simulink model "AMC_BLDC"  (R2023a)
settings: Solver=FixedStepDiscrete  StartTime=0.0  StopTime=10.0  RelTol=1e-3  EnableMultiTasking=on
model workspace (MAT data in the model file):
  AMC_BLDC_Ts = Simulink.Parameter
  AMC_BLDC_Ts.Value = 0.001
  AMC_BLDC_Ts.DataType = 'auto'
  AMC_BLDC_Ts.DocUnits = 's'
  AMC_BLDC_Ts.Complexity = 'real'
  AMC_BLDC_Ts.Dimensions = [1 1]
  ControlFOC_Ts = Simulink.Parameter
  ControlFOC_Ts.Value = 3.65714285714e-05
  ControlFOC_Ts.DataType = 'auto'
  ControlFOC_Ts.DocUnits = 's'
  ControlFOC_Ts.Complexity = 'real'
  ControlFOC_Ts.Dimensions = [1 1]
settings Model: DataDictionary=EmbeddedBoardDD.sldd  Creator=upattacini  LastModifiedBy=mfussi
settings SolverCC: AllowMultiTaskInputOutput=on  ConcurrentTasks=on  AlgebraicLoopSolver=TrustRegion  AutoInsertRateTranBlk=on  InsertRTBMode=Never (minimum delay)
settings DataIOCC: SaveOutput=off  SignalLogging=off  DSMLogging=off  SaveTime=off  ReturnWorkspaceOutputs=off
settings OptimizationCC: DefaultParameterBehavior=Inlined  DefaultUnderspecifiedDataType=single  StrengthReduction=on  PassReuseOutputArgsAs=Individual arguments  ZeroExternalMemoryAtStartup=off  ZeroInternalMemoryAtStartup=off  OptimizeBlockOrder=speed  OptimizationPriority=Speed  OptimizationCustomize=off  MultiThreadedLoops=on  EfficientTunableParamExpr=on
settings DebuggingCC: ParameterPrecisionLossMsg=none  UnconnectedInputMsg=warning  UnconnectedOutputMsg=warning  UnconnectedLineMsg=warning
settings HardwareCC: ProdBitPerPointer=32  ProdBitPerSizeT=32  ProdBitPerPtrDiffT=32  ProdLargestAtomicInteger=Long  ProdLargestAtomicFloat=Double  ProdWordSize=32  ProdHWDeviceType=ARM Compatible->ARM Cortex-M
settings ModelReferenceCC: UpdateModelReferenceTargets=Force  EnableRefExpFcnMdlSchedulingChecks=on  ModelReferenceNumInstancesAllowed=Single
settings SFSimCC: MATLABDynamicMemAlloc=off
settings RTWCC: Description=Embedded Coder  SystemTargetFile=ert.tlc  GenCodeOnly=on  PackageGeneratedCodeAndArtifacts=on  PackageName=AMC_BLDC  TemplateMakefile=ert_default_tmf  TargetLang=C++  DLArmComputeVersion=19.05
settings CodeAppCC: ForceParamTrailComments=on  IgnoreCustomStorageClasses=off  MaxIdLength=60  OperatorAnnotations=on  SimulinkDataObjDesc=on  SFDataObjDesc=on  InsertBlockDesc=on
settings ERTTargetCC: TargetLangStandard=C++03 (ISO)  CodeReplacementLibrary=ARM Cortex-M,iCubTech  GenerateSampleERTMain=on  InlinedParameterPlacement=NonHierarchical  TargetOS=NativeThreadsExample  RootIOFormat=Structure reference  ERTCustomFileTemplate=example_file_process.tlc

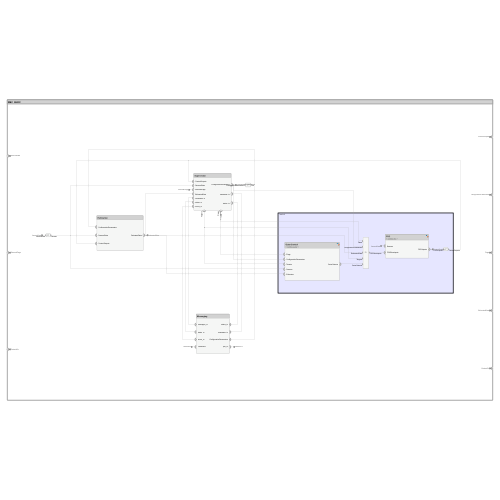
[thumbnail: Simulink's stored preview of the top-level diagram]
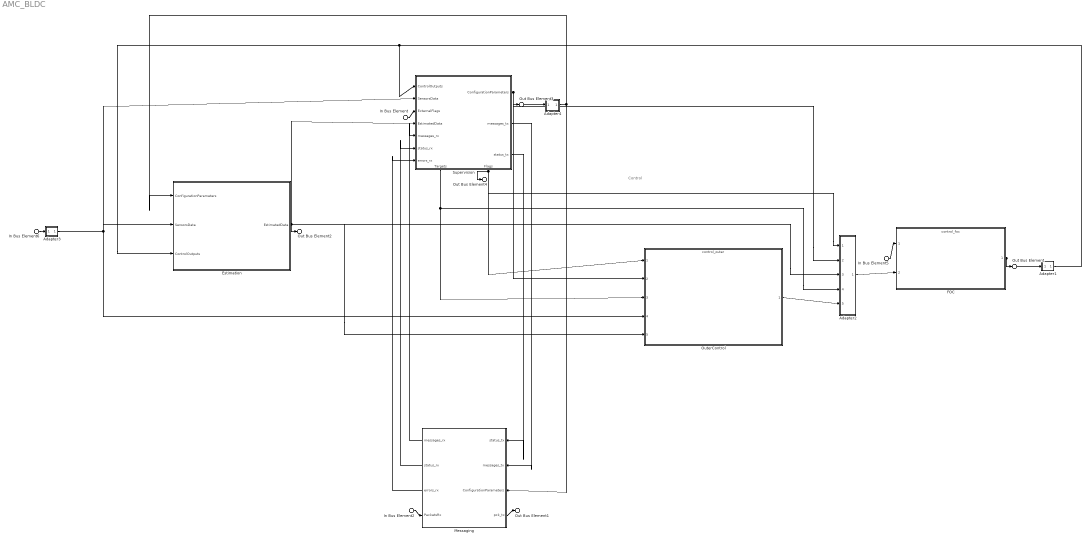
== system AMC_BLDC ==
  note: Control
  In Bus Element5 : Inport  PortName=SensorsData
  In Bus Element6 : Inport  PortName=SensorsData
  In Bus Element : Inport  Port=2  PortName=ExternalFlags
  In Bus Element2 : Inport  Port=3  PortName=PacketsRx
  Adapter1 : Subsystem
      settings: PortSchema="{\"entries\":[{\"content\":{\"margin\":10,\"minimumSpacing\":15,\"sides\":[{\"content\":{\"connectorIds\":[\"In1\"]},\"type\":\"ConnectorPlacement.EquallySpacedRectSide\",\"uuid\":\"3636cd8d-cbd3-4f3a-bfc2-0b6f64e30752\"},{\"content\":{\"connectorIds\":[\"Out1\"],\"side\":\"RIGHT\"},\"type\":\"ConnectorPlacement.EquallySpacedRectSide\",\"uuid\":\"432d5fc1-0f50-4fcc-8edd-5172f2fe1fb1\"},{\"content\":{\"connectorIds\":[],\"side\":\"TOP\"},\"type\":\"ConnectorPlacement.EquallySpacedRectSide\",\"uuid\":\"ba372e81-7918-4711-815e-6864fd5d6a77\"}]},\"type\":\"ConnectorPlacement.EquallySpacedConnector\",\"uuid\":\"ce9b4e59-ddcd-4a55-aad5-bd568399e791\"}],\"packageUris\":[\"http://schema.mathworks.com/mf0/Connector/R2020b\"],\"version\":\"1.0\"}"
  Adapter2 : Subsystem
      settings: PortSchema="{\"entries\":[{\"content\":{\"margin\":10,\"minimumSpacing\":15,\"sides\":[{\"content\":{\"connectorIds\":[\"In1\",\"In2\",\"In3\",\"In4\",\"In5\"]},\"type\":\"ConnectorPlacement.EquallySpacedRectSide\",\"uuid\":\"eaff3585-0474-4235-a4f6-c3e0d182b6aa\"},{\"content\":{\"connectorIds\":[\"Out1\"],\"side\":\"RIGHT\"},\"type\":\"ConnectorPlacement.EquallySpacedRectSide\",\"uuid\":\"c828b82e-1a15-4cb3-9e29-bf61868b0eb2\"},{\"content\":{\"connectorIds\":[],\"side\":\"TOP\"},\"type\":\"ConnectorPlacement.EquallySpacedRectSide\",\"uuid\":\"201fa64a-7527-4a17-8d88-306d6b744e03\"}]},\"type\":\"ConnectorPlacement.EquallySpacedConnector\",\"uuid\":\"604867e8-fac6-4ee4-8cb2-d0c2f12c8ec2\"}],\"packageUris\":[\"http://schema.mathworks.com/mf0/Connector/R2020b\"],\"version\":\"1.0\"}"
  Adapter3 : Subsystem
      settings: PortSchema="{\"entries\":[{\"content\":{\"margin\":10,\"minimumSpacing\":15,\"sides\":[{\"content\":{\"connectorIds\":[\"In1\"]},\"type\":\"ConnectorPlacement.EquallySpacedRectSide\",\"uuid\":\"eaff3585-0474-4235-a4f6-c3e0d182b6aa\"},{\"content\":{\"connectorIds\":[\"Out1\"],\"side\":\"RIGHT\"},\"type\":\"ConnectorPlacement.EquallySpacedRectSide\",\"uuid\":\"c828b82e-1a15-4cb3-9e29-bf61868b0eb2\"},{\"content\":{\"connectorIds\":[],\"side\":\"TOP\"},\"type\":\"ConnectorPlacement.EquallySpacedRectSide\",\"uuid\":\"201fa64a-7527-4a17-8d88-306d6b744e03\"}]},\"type\":\"ConnectorPlacement.EquallySpacedConnector\",\"uuid\":\"604867e8-fac6-4ee4-8cb2-d0c2f12c8ec2\"}],\"packageUris\":[\"http://schema.mathworks.com/mf0/Connector/R2020b\"],\"version\":\"1.0\"}"
  Adapter4 : Subsystem
      settings: PortSchema="{\"entries\":[{\"content\":{\"margin\":10,\"minimumSpacing\":15,\"sides\":[{\"content\":{\"connectorIds\":[\"In1\"]},\"type\":\"ConnectorPlacement.EquallySpacedRectSide\",\"uuid\":\"2422f637-185e-4f0a-81aa-7f0c8ef69ae3\"},{\"content\":{\"connectorIds\":[\"Out1\"],\"side\":\"RIGHT\"},\"type\":\"ConnectorPlacement.EquallySpacedRectSide\",\"uuid\":\"9138eeeb-6d92-412d-9459-f4839966a84c\"},{\"content\":{\"connectorIds\":[],\"side\":\"TOP\"},\"type\":\"ConnectorPlacement.EquallySpacedRectSide\",\"uuid\":\"2441c851-5141-4d9b-bf52-03716abfbc80\"}]},\"type\":\"ConnectorPlacement.EquallySpacedConnector\",\"uuid\":\"4dac98f2-6f5c-4428-8df8-e9410164b098\"}],\"packageUris\":[\"http://schema.mathworks.com/mf0/Connector/R2020b\"],\"version\":\"1.0\"}"
  Estimation : Subsystem
      settings: PortSchema="{\"entries\":[{\"content\":{\"headerSize\":26,\"margin\":15,\"minimumSpacing\":25,\"sides\":[{\"content\":{\"connectorIds\":[\"In1\",\"In2\",\"In3\"]},\"type\":\"ConnectorPlacement.EquallySpacedRectSide\",\"uuid\":\"aa685b80-0b4c-4380-a51a-9e8b188668b2\"},{\"content\":{\"connectorIds\":[\"Out1\"],\"side\":\"RIGHT\"},\"type\":\"ConnectorPlacement.EquallySpacedRectSide\",\"uuid\":\"f0a2eecf-364b-49e3-8f56-34a9b5626df1\"},{\"content\":{\"connectorIds\":[],\"side\":\"TOP\"},\"type\":\"ConnectorPlacement.EquallySpacedRectSide\",\"uuid\":\"7dba8d43-602c-42b6-8ef7-63524ab126d1\"}]},\"type\":\"ConnectorPlacement.EquallySpacedConnector\",\"uuid\":\"2c3a6225-3f46-4b42-9094-6f425be46a6a\"}],\"packageUris\":[\"http://schema.mathworks.com/mf0/Connector/R2020b\"],\"version\":\"1.0\"}"
  FOC : ModelReference  ModelNameDialog=control_foc  SimulationMode=Normal  ModelReferenceVersion=5.13
      settings: PortSchema="{\"entries\":[{\"content\":{\"headerSize\":38,\"margin\":15,\"minimumSpacing\":25,\"sides\":[{\"content\":{\"connectorIds\":[\"In1\",\"In2\"]},\"type\":\"ConnectorPlacement.EquallySpacedRectSide\",\"uuid\":\"55fc5d39-1c77-43ba-92cf-c46a3d0b9743\"},{\"content\":{\"connectorIds\":[\"Out1\"],\"side\":\"RIGHT\"},\"type\":\"ConnectorPlacement.EquallySpacedRectSide\",\"uuid\":\"069c7079-ecb9-46eb-b98e-d35431f03a55\"},{\"content\":{\"connectorIds\":[],\"side\":\"TOP\"},\"type\":\"ConnectorPlacement.EquallySpacedRectSide\",\"uuid\":\"f3e493a2-5661-4841-b7c0-29b471d59bca\"}]},\"type\":\"ConnectorPlacement.EquallySpacedConnector\",\"uuid\":\"e5d0bfdd-5add-4be0-a4f6-a6948864cef2\"}],\"packageUris\":[\"http://schema.mathworks.com/mf0/Connector/R2020b\"],\"version\":\"1.0\"}"
  Messaging : Subsystem
      settings: PortSchema="{\"entries\":[{\"content\":{\"headerSize\":26,\"margin\":15,\"minimumSpacing\":25,\"sides\":[{\"content\":{\"connectorIds\":[\"Out2\",\"Out3\",\"Out4\",\"In1\"]},\"type\":\"ConnectorPlacement.EquallySpacedRectSide\",\"uuid\":\"2148a9ca-a041-4019-8738-bc30807315dc\"},{\"content\":{\"connectorIds\":[\"In4\",\"In2\",\"In3\",\"Out1\"],\"side\":\"RIGHT\"},\"type\":\"ConnectorPlacement.EquallySpacedRectSide\",\"uuid\":\"d2884f22-8c53-43de-b638-02974377300f\"},{\"content\":{\"connectorIds\":[],\"side\":\"TOP\"},\"type\":\"ConnectorPlacement.EquallySpacedRectSide\",\"uuid\":\"0563c894-934a-48e6-bdf6-cacba4ee5b45\"},{\"content\":{\"connectorIds\":[],\"side\":\"BOTTOM\"},\"type\":\"ConnectorPlacement.EquallySpacedRectSide\",\"uuid\":\"9d0264c3-5ca4-4a71-92f0-4ebcad17af76\"}]},\"type\":\"ConnectorPlacement.EquallySpacedConnector\",\"uuid\":\"aceedaa9-7f20-49f1-93cc-8d7be38f8964\"}],\"packageUris\":[\"http://schema.mathworks.com/mf0/Connector/R2020b\"],\"version\":\"1.0\"}"
  OuterControl : ModelReference  ModelNameDialog=control_outer.slx  SimulationMode=Normal  ModelReferenceVersion=5.5
      settings: PortSchema="{\"entries\":[{\"content\":{\"headerSize\":38,\"margin\":15,\"minimumSpacing\":25,\"sides\":[{\"content\":{\"connectorIds\":[\"In1\",\"In2\",\"In3\",\"In4\",\"In5\"]},\"type\":\"ConnectorPlacement.EquallySpacedRectSide\",\"uuid\":\"2148a9ca-a041-4019-8738-bc30807315dc\"},{\"content\":{\"connectorIds\":[\"Out1\"],\"side\":\"RIGHT\"},\"type\":\"ConnectorPlacement.EquallySpacedRectSide\",\"uuid\":\"d2884f22-8c53-43de-b638-02974377300f\"},{\"content\":{\"connectorIds\":[],\"side\":\"TOP\"},\"type\":\"ConnectorPlacement.EquallySpacedRectSide\",\"uuid\":\"0563c894-934a-48e6-bdf6-cacba4ee5b45\"}]},\"type\":\"ConnectorPlacement.EquallySpacedConnector\",\"uuid\":\"aceedaa9-7f20-49f1-93cc-8d7be38f8964\"}],\"packageUris\":[\"http://schema.mathworks.com/mf0/Connector/R2020b\"],\"version\":\"1.0\"}"
  Supervision : Subsystem
      settings: PortSchema="{\"entries\":[{\"content\":{\"headerSize\":26,\"margin\":15,\"minimumSpacing\":25,\"sides\":[{\"content\":{\"connectorIds\":[\"In7\",\"In1\",\"In3\",\"In2\",\"In4\",\"In5\",\"In6\"]},\"type\":\"ConnectorPlacement.EquallySpacedRectSide\",\"uuid\":\"d8d95745-d05d-4d59-a714-83471558f722\"},{\"content\":{\"connectorIds\":[\"Out5\",\"Out2\",\"Out3\"],\"side\":\"RIGHT\"},\"type\":\"ConnectorPlacement.EquallySpacedRectSide\",\"uuid\":\"f4a8c463-a5d8-439b-a3c8-9fd952511ae5\"},{\"content\":{\"connectorIds\":[],\"side\":\"TOP\"},\"type\":\"ConnectorPlacement.EquallySpacedRectSide\",\"uuid\":\"4f11964b-14d9-4acd-b1b8-e8b82e3000f1\"},{\"content\":{\"connectorIds\":[\"Out1\",\"Out4\"],\"side\":\"BOTTOM\"},\"type\":\"ConnectorPlacement.EquallySpacedRectSide\",\"uuid\":\"505ec373-588b-4be2-9f68-334cbdc0ac1c\"},{\"content\":{\"connectorIds\":[],\"side\":\"HIDDEN\"},\"type\":\"ConnectorPlacement.EquallySpacedRectSide\",\"uuid\":\"02bfd962-06b7-4437-adb6-71eb1824f80b\"}]},\"type\":\"ConnectorPlacement.EquallySpacedConnector\",\"uuid\":\"2e282e5b-c538-411e-81ed-553352dd5c9d\"}],\"packageUris\":[\"http://schema.mathworks.com/mf0/Connector/R2020b\"],\"version\":\"1.0\"}"
  Out Bus Element : Outport  PortName=ControlOutputs
  Out Bus Element3 : Outport  Port=2  PortName=ConfigurationParameters
  Out Bus Element4 : Outport  Port=3  PortName=Flags
  Out Bus Element2 : Outport  Port=4  PortName=EstimatedData
  Out Bus Element1 : Outport  Port=5  PortName=PacketsTx
  wires:
  Supervision/5(ConfigurationParameters) -> Adapter2/2(ConfigurationParameters), OuterControl/2, Out Bus Element3/1, Adapter4/1(ConfigurationParameters)
  In Bus Element2/1 -> Messaging/1(PacketsRx)
  Messaging/2(messages_rx) -> Supervision/4(messages_rx)
  Messaging/3(status_rx) -> Supervision/5(status_rx)
  Messaging/4(errors_rx) -> Supervision/6(errors_rx)
  Estimation/1(EstimatedData) -> Supervision/2(EstimatedData), Out Bus Element2/1, OuterControl/5, Adapter2/3(EstimatedData)
  FOC/1 -> Out Bus Element/1, Adapter1/1(FOCOutputs)
  Adapter1/1(ControlOutputs) -> Supervision/7(ControlOutputs), Estimation/3(ControlOutputs)
  Adapter2/1(FOCSlowInputs) -> FOC/2
  In Bus Element5/1 -> FOC/1
  OuterControl/1 -> Adapter2/5(OuterOutputs)
  In Bus Element6/1 -> Adapter3/1(SensorsData)
  Adapter3/1(Sensors) -> OuterControl/4, Supervision/1(SensorsData), Estimation/2(SensorsData)
  Supervision/2(messages_tx) -> Messaging/2(messages_tx)
  Supervision/3(status_tx) -> Messaging/4(status_tx)
  Supervision/4(Flags) -> OuterControl/1, Adapter2/1(Flags), Out Bus Element4/1
  Supervision/1(Targets) -> Adapter2/4(Targets), OuterControl/3
  In Bus Element/1 -> Supervision/3(ExternalFlags)
  Messaging/1(pck_tx) -> Out Bus Element1/1
  Adapter4/1(Out) -> Messaging/3(ConfigurationParameters), Estimation/1(ConfigurationParameters)

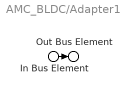
== system AMC_BLDC/Adapter1 ==
  In Bus Element : Inport  PortName=FOCOutputs
  Out Bus Element : Outport  PortName=ControlOutputs
  wires:
  In Bus Element/1 -> Out Bus Element/1

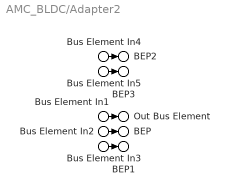
== system AMC_BLDC/Adapter2 ==
  Bus Element In1 : Inport  PortName=Flags
  Bus Element In2 : Inport  Port=2  PortName=ConfigurationParameters
  Bus Element In3 : Inport  Port=3  PortName=EstimatedData
  Bus Element In4 : Inport  Port=4  PortName=Targets
  Bus Element In5 : Inport  Port=5  PortName=OuterOutputs
  Out Bus Element : Outport  PortName=FOCSlowInputs  Element=flags
  BEP : Outport  PortName=FOCSlowInputs  Element=configurationparameters
  BEP1 : Outport  PortName=FOCSlowInputs  Element=estimateddata
  BEP2 : Outport  PortName=FOCSlowInputs  Element=targets
  BEP3 : Outport  PortName=FOCSlowInputs  Element=controlouteroutputs
  wires:
  Bus Element In1/1 -> Out Bus Element/1
  Bus Element In2/1 -> BEP/1
  Bus Element In3/1 -> BEP1/1
  Bus Element In4/1 -> BEP2/1
  Bus Element In5/1 -> BEP3/1

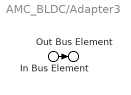
== system AMC_BLDC/Adapter3 ==
  In Bus Element : Inport  PortName=SensorsData
  Out Bus Element : Outport  PortName=Sensors
  wires:
  In Bus Element/1 -> Out Bus Element/1

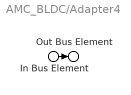
== system AMC_BLDC/Adapter4 ==
  In Bus Element : Inport  PortName=ConfigurationParameters
  Out Bus Element : Outport  PortName=Out
  wires:
  In Bus Element/1 -> Out Bus Element/1

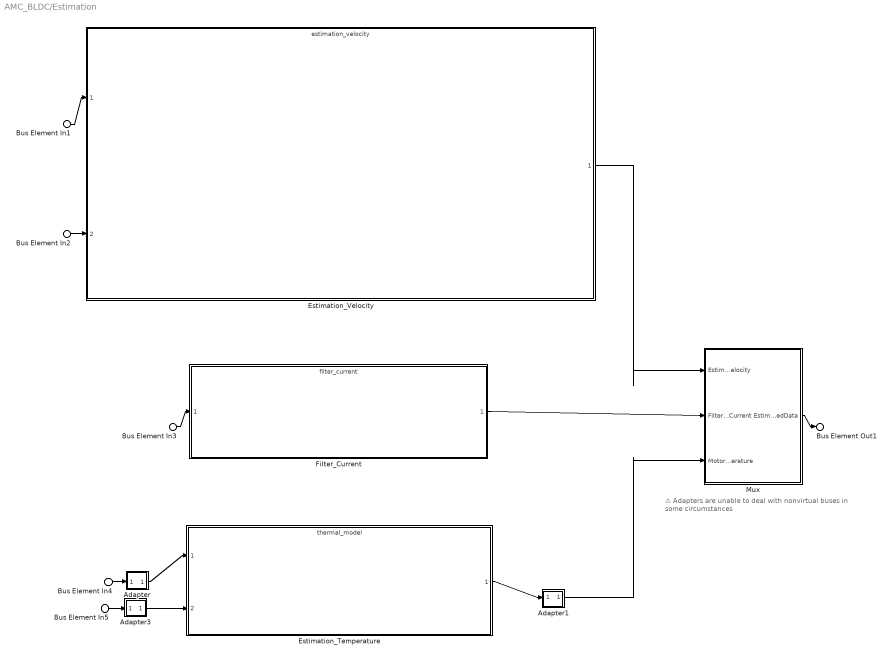
== system AMC_BLDC/Estimation ==
  note: ⚠️ Adapters are unable to deal with nonvirtual buses
      | in some circumstances
  Bus Element In2 : Inport  PortName=ConfigurationParameters
  Bus Element In5 : Inport  PortName=ConfigurationParameters
  Bus Element In1 : Inport  Port=2  PortName=SensorsData
  Bus Element In3 : Inport  Port=3  PortName=ControlOutputs
  Bus Element In4 : Inport  Port=3  PortName=ControlOutputs
  Adapter : Subsystem
      settings: PortSchema="{\"entries\":[{\"content\":{\"margin\":10,\"minimumSpacing\":15,\"sides\":[{\"content\":{\"connectorIds\":[\"In1\"]},\"type\":\"ConnectorPlacement.EquallySpacedRectSide\",\"uuid\":\"1533dfbf-f117-431b-b1c8-daccd425eade\"},{\"content\":{\"connectorIds\":[\"Out1\"],\"side\":\"RIGHT\"},\"type\":\"ConnectorPlacement.EquallySpacedRectSide\",\"uuid\":\"2b2dea55-3ac8-49ca-9e1e-82c04720b164\"},{\"content\":{\"side\":\"TOP\"},\"type\":\"ConnectorPlacement.EquallySpacedRectSide\",\"uuid\":\"bef9b798-8ddf-4a62-a2af-1ba3ae2c0941\"}]},\"type\":\"ConnectorPlacement.EquallySpacedConnector\",\"uuid\":\"f1f6f3c3-ef56-4107-bd04-a8a31aeae809\"}],\"packageUris\":[\"http://schema.mathworks.com/mf0/Connector/R2020b\"],\"version\":\"1.0\"}"
  Adapter1 : Subsystem
      settings: PortSchema="{\"entries\":[{\"content\":{\"margin\":10,\"minimumSpacing\":15,\"sides\":[{\"content\":{\"connectorIds\":[\"In1\"]},\"type\":\"ConnectorPlacement.EquallySpacedRectSide\",\"uuid\":\"bd134203-0b3b-4af9-96b7-dab0f59a0c1f\"},{\"content\":{\"connectorIds\":[\"Out1\"],\"side\":\"RIGHT\"},\"type\":\"ConnectorPlacement.EquallySpacedRectSide\",\"uuid\":\"18b3782d-59db-4de9-a61f-4faacc42cb35\"},{\"content\":{\"side\":\"TOP\"},\"type\":\"ConnectorPlacement.EquallySpacedRectSide\",\"uuid\":\"5978c1b5-2fbd-45fe-b5e8-51aa489915dc\"}]},\"type\":\"ConnectorPlacement.EquallySpacedConnector\",\"uuid\":\"defdca45-a432-4484-981c-f193c096ad07\"}],\"packageUris\":[\"http://schema.mathworks.com/mf0/Connector/R2020b\"],\"version\":\"1.0\"}"
  Adapter3 : Subsystem
      settings: PortSchema="{\"entries\":[{\"content\":{\"margin\":10,\"minimumSpacing\":15,\"sides\":[{\"content\":{\"connectorIds\":[\"In1\"]},\"type\":\"ConnectorPlacement.EquallySpacedRectSide\",\"uuid\":\"1533dfbf-f117-431b-b1c8-daccd425eade\"},{\"content\":{\"connectorIds\":[\"Out1\"],\"side\":\"RIGHT\"},\"type\":\"ConnectorPlacement.EquallySpacedRectSide\",\"uuid\":\"2b2dea55-3ac8-49ca-9e1e-82c04720b164\"},{\"content\":{\"side\":\"TOP\"},\"type\":\"ConnectorPlacement.EquallySpacedRectSide\",\"uuid\":\"bef9b798-8ddf-4a62-a2af-1ba3ae2c0941\"}]},\"type\":\"ConnectorPlacement.EquallySpacedConnector\",\"uuid\":\"f1f6f3c3-ef56-4107-bd04-a8a31aeae809\"}],\"packageUris\":[\"http://schema.mathworks.com/mf0/Connector/R2020b\"],\"version\":\"1.0\"}"
  Estimation_Temperature : ModelReference  ModelNameDialog=thermal_model  SimulationMode=Normal  ModelReferenceVersion=5.21
      settings: PortSchema="{\"entries\":[{\"content\":{\"headerSize\":38,\"margin\":15,\"minimumSpacing\":25,\"sides\":[{\"content\":{\"connectorIds\":[\"In1\",\"In2\"]},\"type\":\"ConnectorPlacement.EquallySpacedRectSide\",\"uuid\":\"bd134203-0b3b-4af9-96b7-dab0f59a0c1f\"},{\"content\":{\"connectorIds\":[\"Out1\"],\"side\":\"RIGHT\"},\"type\":\"ConnectorPlacement.EquallySpacedRectSide\",\"uuid\":\"18b3782d-59db-4de9-a61f-4faacc42cb35\"},{\"content\":{\"side\":\"TOP\"},\"type\":\"ConnectorPlacement.EquallySpacedRectSide\",\"uuid\":\"5978c1b5-2fbd-45fe-b5e8-51aa489915dc\"}]},\"type\":\"ConnectorPlacement.EquallySpacedConnector\",\"uuid\":\"defdca45-a432-4484-981c-f193c096ad07\"}],\"packageUris\":[\"http://schema.mathworks.com/mf0/Connector/R2020b\"],\"version\":\"1.0\"}"
  Estimation_Velocity : ModelReference  ModelNameDialog=estimation_velocity  SimulationMode=Normal  ModelReferenceVersion=5.1
      settings: PortSchema="{\"entries\":[{\"content\":{\"headerSize\":38,\"margin\":15,\"minimumSpacing\":25,\"sides\":[{\"content\":{\"connectorIds\":[\"In1\",\"In2\"]},\"type\":\"ConnectorPlacement.EquallySpacedRectSide\",\"uuid\":\"c20bbcf3-caa1-470b-9404-350c64a63ecb\"},{\"content\":{\"connectorIds\":[\"Out1\"],\"side\":\"RIGHT\"},\"type\":\"ConnectorPlacement.EquallySpacedRectSide\",\"uuid\":\"349ddba8-7d90-466d-b62e-3b2add687930\"},{\"content\":{\"connectorIds\":[],\"side\":\"TOP\"},\"type\":\"ConnectorPlacement.EquallySpacedRectSide\",\"uuid\":\"ab4ae875-bf4c-4a6b-8d97-80279b03fcf4\"}]},\"type\":\"ConnectorPlacement.EquallySpacedConnector\",\"uuid\":\"748f1452-f2e6-4654-80a3-86ed1345138b\"}],\"packageUris\":[\"http://schema.mathworks.com/mf0/Connector/R2020b\"],\"version\":\"1.0\"}"
  Filter_Current : ModelReference  ModelNameDialog=filter_current  SimulationMode=Normal  ModelReferenceVersion=5.1
      settings: PortSchema="{\"entries\":[{\"content\":{\"headerSize\":38,\"margin\":15,\"minimumSpacing\":25,\"sides\":[{\"content\":{\"connectorIds\":[\"In1\"]},\"type\":\"ConnectorPlacement.EquallySpacedRectSide\",\"uuid\":\"55cf2034-b9d8-4a6c-92aa-69b36d7513a6\"},{\"content\":{\"connectorIds\":[\"Out1\"],\"side\":\"RIGHT\"},\"type\":\"ConnectorPlacement.EquallySpacedRectSide\",\"uuid\":\"f8b242ba-9027-4fc8-afba-27f3d06cf2e2\"},{\"content\":{\"connectorIds\":[],\"side\":\"TOP\"},\"type\":\"ConnectorPlacement.EquallySpacedRectSide\",\"uuid\":\"6b682352-097d-447e-888e-81a3c9658083\"}]},\"type\":\"ConnectorPlacement.EquallySpacedConnector\",\"uuid\":\"9bf2e5ad-6e16-4309-91f6-03add447b5ae\"}],\"packageUris\":[\"http://schema.mathworks.com/mf0/Connector/R2020b\"],\"version\":\"1.0\"}"
  Mux : Subsystem
      settings: PortSchema="{\"entries\":[{\"content\":{\"headerSize\":26,\"margin\":15,\"minimumSpacing\":25,\"sides\":[{\"content\":{\"connectorIds\":[\"In1\",\"In2\",\"In3\"]},\"type\":\"ConnectorPlacement.EquallySpacedRectSide\",\"uuid\":\"55cf2034-b9d8-4a6c-92aa-69b36d7513a6\"},{\"content\":{\"connectorIds\":[\"Out1\"],\"side\":\"RIGHT\"},\"type\":\"ConnectorPlacement.EquallySpacedRectSide\",\"uuid\":\"f8b242ba-9027-4fc8-afba-27f3d06cf2e2\"},{\"content\":{\"side\":\"TOP\"},\"type\":\"ConnectorPlacement.EquallySpacedRectSide\",\"uuid\":\"6b682352-097d-447e-888e-81a3c9658083\"}]},\"type\":\"ConnectorPlacement.EquallySpacedConnector\",\"uuid\":\"9bf2e5ad-6e16-4309-91f6-03add447b5ae\"}],\"packageUris\":[\"http://schema.mathworks.com/mf0/Connector/R2020b\"],\"version\":\"1.0\"}"
  Bus Element Out1 : Outport  PortName=EstimatedData
  wires:
  Bus Element In1/1 -> Estimation_Velocity/1
  Bus Element In2/1 -> Estimation_Velocity/2
  Estimation_Velocity/1 -> Mux/1(EstimatedVelocity)
  Filter_Current/1 -> Mux/2(FilteredCurrent)
  Mux/1(EstimatedData) -> Bus Element Out1/1
  Adapter1/1(Out) -> Mux/3(MotorTemperature)
  Bus Element In3/1 -> Filter_Current/1
  Estimation_Temperature/1 -> Adapter1/1(In)
  Adapter/1(Out) -> Estimation_Temperature/1
  Bus Element In4/1 -> Adapter/1(ControlOutputs)
  Bus Element In5/1 -> Adapter3/1(ConfigurationParameters)
  Adapter3/1(Out) -> Estimation_Temperature/2

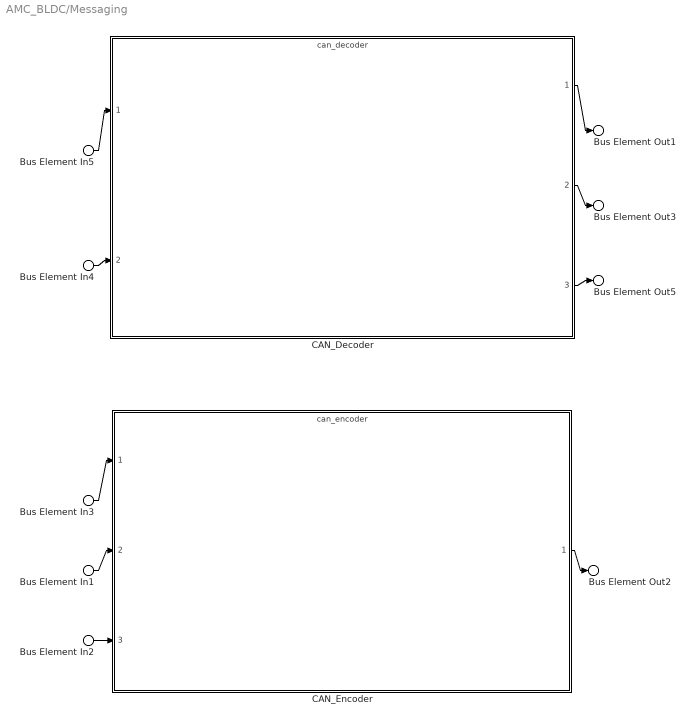
== system AMC_BLDC/Messaging ==
  Bus Element In5 : Inport  PortName=PacketsRx
  Bus Element In3 : Inport  Port=2  PortName=messages_tx
  Bus Element In2 : Inport  Port=3  PortName=ConfigurationParameters
  Bus Element In4 : Inport  Port=3  PortName=ConfigurationParameters
  Bus Element In1 : Inport  Port=4  PortName=status_tx
  CAN_Decoder : ModelReference  ModelNameDialog=can_decoder  SimulationMode=Normal  ModelReferenceVersion=5.0
      settings: PortSchema="{\"entries\":[{\"content\":{\"headerSize\":38,\"margin\":15,\"minimumSpacing\":25,\"sides\":[{\"content\":{\"connectorIds\":[\"In1\",\"In2\"]},\"type\":\"ConnectorPlacement.EquallySpacedRectSide\",\"uuid\":\"b2b94824-c700-4373-91d8-47add34cc094\"},{\"content\":{\"connectorIds\":[\"Out1\",\"Out2\",\"Out3\"],\"side\":\"RIGHT\"},\"type\":\"ConnectorPlacement.EquallySpacedRectSide\",\"uuid\":\"93c2845f-b99b-4543-8e08-c46ac526332e\"},{\"content\":{\"connectorIds\":[],\"side\":\"TOP\"},\"type\":\"ConnectorPlacement.EquallySpacedRectSide\",\"uuid\":\"58bbde8c-049b-4e4b-9306-530fa2daad17\"}]},\"type\":\"ConnectorPlacement.EquallySpacedConnector\",\"uuid\":\"2d51588d-c4d7-43f4-87c2-9173ed7811d6\"}],\"packageUris\":[\"http://schema.mathworks.com/mf0/Connector/R2020b\"],\"version\":\"1.0\"}"
  CAN_Encoder : ModelReference  ModelNameDialog=can_encoder  SimulationMode=Normal  ModelReferenceVersion=5.0
      settings: PortSchema="{\"entries\":[{\"content\":{\"headerSize\":38,\"margin\":15,\"minimumSpacing\":25,\"sides\":[{\"content\":{\"connectorIds\":[\"In1\",\"In2\",\"In3\"]},\"type\":\"ConnectorPlacement.EquallySpacedRectSide\",\"uuid\":\"6f4b08cd-f6c5-49bf-b1cb-2cd7d6623be6\"},{\"content\":{\"connectorIds\":[\"Out1\"],\"side\":\"RIGHT\"},\"type\":\"ConnectorPlacement.EquallySpacedRectSide\",\"uuid\":\"50a4d36e-deb5-40a6-b950-d37a57b313ee\"},{\"content\":{\"connectorIds\":[],\"side\":\"TOP\"},\"type\":\"ConnectorPlacement.EquallySpacedRectSide\",\"uuid\":\"f26608a5-c459-46f7-8e1f-f1e374dcdcf6\"}]},\"type\":\"ConnectorPlacement.EquallySpacedConnector\",\"uuid\":\"e591c604-78a1-48e3-93c5-357c40d96f0b\"}],\"packageUris\":[\"http://schema.mathworks.com/mf0/Connector/R2020b\"],\"version\":\"1.0\"}"
  Bus Element Out2 : Outport  PortName=pck_tx
  Bus Element Out1 : Outport  Port=2  PortName=messages_rx
  Bus Element Out3 : Outport  Port=3  PortName=status_rx
  Bus Element Out5 : Outport  Port=4  PortName=errors_rx
  wires:
  CAN_Decoder/1 -> Bus Element Out1/1
  CAN_Decoder/2 -> Bus Element Out3/1
  CAN_Decoder/3 -> Bus Element Out5/1
  Bus Element In3/1 -> CAN_Encoder/1
  Bus Element In1/1 -> CAN_Encoder/2
  CAN_Encoder/1 -> Bus Element Out2/1
  Bus Element In5/1 -> CAN_Decoder/1
  Bus Element In2/1 -> CAN_Encoder/3
  Bus Element In4/1 -> CAN_Decoder/2

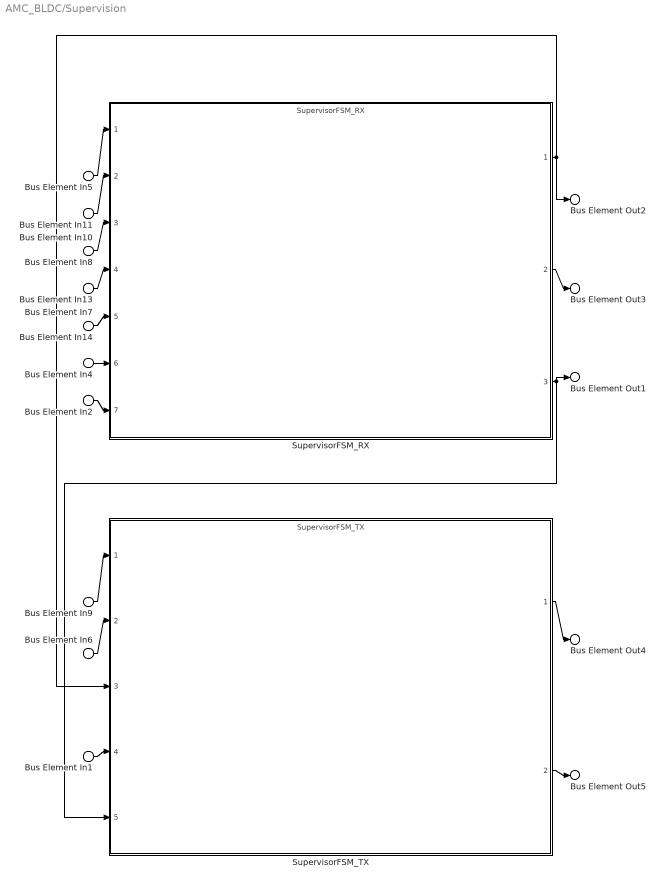
== system AMC_BLDC/Supervision ==
  Bus Element In9 : Inport  PortName=SensorsData
  Bus Element In5 : Inport  PortName=SensorsData
  Bus Element In8 : Inport  Port=2  PortName=EstimatedData
  Bus Element In14 : Inport  Port=2  PortName=EstimatedData
  Bus Element In6 : Inport  Port=2  PortName=EstimatedData
  Bus Element In11 : Inport  Port=3  PortName=ExternalFlags
  Bus Element In7 : Inport  Port=4  PortName=messages_rx
  Bus Element In13 : Inport  Port=4  PortName=messages_rx
  Bus Element In4 : Inport  Port=5  PortName=status_rx
  Bus Element In2 : Inport  Port=6  PortName=errors_rx
  Bus Element In10 : Inport  Port=7  PortName=ControlOutputs
  Bus Element In1 : Inport  Port=7  PortName=ControlOutputs
  SupervisorFSM_RX : ModelReference  ModelNameDialog=SupervisorFSM_RX.slx  SimulationMode=Normal  ModelReferenceVersion=6.22
      settings: PortSchema="{\"entries\":[{\"content\":{\"headerSize\":38,\"margin\":15,\"minimumSpacing\":25,\"sides\":[{\"content\":{\"connectorIds\":[\"In1\",\"In2\",\"In3\",\"In4\",\"In5\",\"In6\",\"In7\"]},\"type\":\"ConnectorPlacement.EquallySpacedRectSide\",\"uuid\":\"4aedf767-9c1b-4c88-bc72-7777321bcd41\"},{\"content\":{\"connectorIds\":[\"Out1\",\"Out2\",\"Out3\"],\"side\":\"RIGHT\"},\"type\":\"ConnectorPlacement.EquallySpacedRectSide\",\"uuid\":\"aee88cc0-e097-47ae-97af-9ad4a0a9b7bf\"},{\"content\":{\"connectorIds\":[],\"side\":\"TOP\"},\"type\":\"ConnectorPlacement.EquallySpacedRectSide\",\"uuid\":\"173fabf3-9ac1-4c2f-9d1c-2c077518d79f\"},{\"content\":{\"connectorIds\":[],\"side\":\"HIDDEN\"},\"type\":\"ConnectorPlacement.EquallySpacedRectSide\",\"uuid\":\"c63b284f-1c4e-4f1a-bde6-4ce5f749d319\"}]},\"type\":\"ConnectorPlacement.EquallySpacedConnector\",\"uuid\":\"40fdf982-cc0d-4196-8efc-330d112bcb29\"}],\"packageUris\":[\"http://schema.mathworks.com/mf0/Connector/R2020b\"],\"version\":\"1.0\"}"
  SupervisorFSM_TX : ModelReference  ModelNameDialog=SupervisorFSM_TX.slx  SimulationMode=Normal  ModelReferenceVersion=6.1
      settings: PortSchema="{\"entries\":[{\"content\":{\"headerSize\":38,\"margin\":15,\"minimumSpacing\":25,\"sides\":[{\"content\":{\"connectorIds\":[\"In1\",\"In2\",\"In3\",\"In4\",\"In5\"]},\"type\":\"ConnectorPlacement.EquallySpacedRectSide\",\"uuid\":\"4aedf767-9c1b-4c88-bc72-7777321bcd41\"},{\"content\":{\"connectorIds\":[\"Out1\",\"Out2\"],\"side\":\"RIGHT\"},\"type\":\"ConnectorPlacement.EquallySpacedRectSide\",\"uuid\":\"aee88cc0-e097-47ae-97af-9ad4a0a9b7bf\"},{\"content\":{\"connectorIds\":[],\"side\":\"TOP\"},\"type\":\"ConnectorPlacement.EquallySpacedRectSide\",\"uuid\":\"173fabf3-9ac1-4c2f-9d1c-2c077518d79f\"},{\"content\":{\"connectorIds\":[],\"side\":\"HIDDEN\"},\"type\":\"ConnectorPlacement.EquallySpacedRectSide\",\"uuid\":\"c63b284f-1c4e-4f1a-bde6-4ce5f749d319\"}]},\"type\":\"ConnectorPlacement.EquallySpacedConnector\",\"uuid\":\"40fdf982-cc0d-4196-8efc-330d112bcb29\"}],\"packageUris\":[\"http://schema.mathworks.com/mf0/Connector/R2020b\"],\"version\":\"1.0\"}"
  Bus Element Out3 : Outport  PortName=Targets
  Bus Element Out4 : Outport  Port=2  PortName=messages_tx
  Bus Element Out5 : Outport  Port=3  PortName=status_tx
  Bus Element Out2 : Outport  Port=4  PortName=Flags
  Bus Element Out1 : Outport  Port=5  PortName=ConfigurationParameters
  wires:
  Bus Element In11/1 -> SupervisorFSM_RX/2
  Bus Element In13/1 -> SupervisorFSM_RX/4
  Bus Element In14/1 -> SupervisorFSM_RX/5
  Bus Element In4/1 -> SupervisorFSM_RX/6
  Bus Element In2/1 -> SupervisorFSM_RX/7
  SupervisorFSM_RX/2 -> Bus Element Out3/1
  SupervisorFSM_RX/3 -> SupervisorFSM_TX/5, Bus Element Out1/1
  SupervisorFSM_TX/1 -> Bus Element Out4/1
  Bus Element In6/1 -> SupervisorFSM_TX/2
  Bus Element In9/1 -> SupervisorFSM_TX/1
  SupervisorFSM_RX/1 -> SupervisorFSM_TX/3, Bus Element Out2/1
  SupervisorFSM_TX/2 -> Bus Element Out5/1
  Bus Element In10/1 -> SupervisorFSM_RX/3
  Bus Element In1/1 -> SupervisorFSM_TX/4
  Bus Element In5/1 -> SupervisorFSM_RX/1

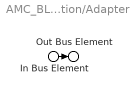
== system AMC_BLDC/Estimation/Adapter ==
  In Bus Element : Inport  PortName=ControlOutputs
  Out Bus Element : Outport  PortName=Out
  wires:
  In Bus Element/1 -> Out Bus Element/1

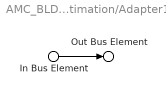
== system AMC_BLDC/Estimation/Adapter1 ==
  In Bus Element : Inport  PortName=In
  Out Bus Element : Outport  PortName=Out
  wires:
  In Bus Element/1 -> Out Bus Element/1

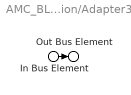
== system AMC_BLDC/Estimation/Adapter3 ==
  In Bus Element : Inport  PortName=ConfigurationParameters
  Out Bus Element : Outport  PortName=Out
  wires:
  In Bus Element/1 -> Out Bus Element/1

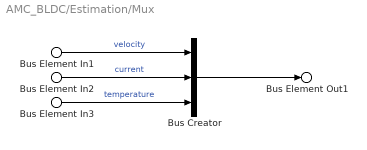
== system AMC_BLDC/Estimation/Mux ==
  Bus Element In1 : Inport  PortName=EstimatedVelocity
  Bus Element In2 : Inport  Port=2  PortName=FilteredCurrent
  Bus Element In3 : Inport  Port=3  PortName=MotorTemperature
  Bus Creator : BusCreator  Inputs=3  OutDataTypeStr=Bus: EstimatedData  NonVirtualBus=on
      settings: InheritFromInputs=off
  Bus Element Out1 : Outport  PortName=EstimatedData
  wires:
  Bus Creator/1 -> Bus Element Out1/1
  Bus Element In1/1 -> Bus Creator/1  "velocity"
  Bus Element In2/1 -> Bus Creator/2  "current"
  Bus Element In3/1 -> Bus Creator/3  "temperature"
